simulink model "simulink_main"  (R2020b)
settings: Solver=FixedStepAuto  StartTime=0.0  StopTime=simTime  FixedStep=simulationStepTime  MaxStep=simulationStepTime  RelTol=1e-3
values from neighbouring files (symbols this model uses):
  link1MaxThreshold = 0    [main_CDTA.m]
  link1MinThreshold = 1    [main_CDTA.m]
undefined symbols (not defined in the file or in its folder): delayCPE1Controller1, delayCPE2Controller1, processingTimeCPEUpdate, processTimeController1, processTimeCPE1MonitoringInfo
settings Model: Creator=carmi  LastModifiedBy=carmi
settings DataIOCC: LimitDataPoints=on  SaveOutput=off  SaveTime=off  ReturnWorkspaceOutputs=off
settings OptimizationCC: BooleanDataType=off  DefaultParameterBehavior=Inlined  LocalBlockOutputs=off  LifeSpan=inf
settings DebuggingCC: AlgebraicLoopMsg=error  SingleTaskRateTransMsg=error  AllowSymbolicDim=off  SFUnexpectedBacktrackingDiag=warning  SFNoUnconditionalDefaultTransitionDiag=warning  SFExecutionAtInitializationDiag=none  ArithmeticOperatorsInVariantConditions=warning
settings SFSimCC: SimUseLocalCustomCode=off  CustomCodeUndefinedFunction=UseInterfaceOnly
settings RTWCC: RTWUseLocalCustomCode=off
settings CodeAppCC: StateflowObjectComments=on
settings GRTTargetCC: TargetLangStandard=C89/C90 (ANSI)
settings ConfigComp: CovMetricSettings=dw  CovSaveCumulativeToWorkspaceVar=on  CovSaveSingleToWorkspaceVar=on  CovExternalEMLEnable=off  CovSFcnEnable=off

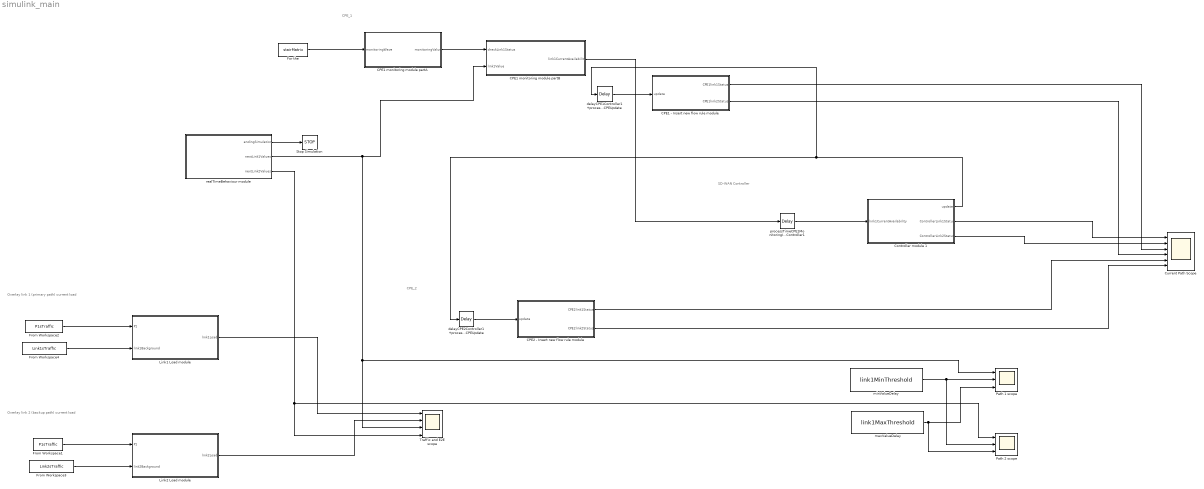
== system simulink_main ==
  note: SD-WAN Controller
  note: Overlay link 2 (backup path) current load
  note: CPE_1
  note: CPE_2
  note: Overlay link 1 (primary path) current load
  CPE1 - Insert new flow rule module : MATLAB Function  TreatAsAtomicUnit=on
  CPE1 monitoring module partA : MATLAB Function  TreatAsAtomicUnit=on
  CPE1 monitoring module partB : MATLAB Function  TreatAsAtomicUnit=on
  CPE2 - Insert new flow rule module : MATLAB Function  TreatAsAtomicUnit=on
  "Controller module 1 " : MATLAB Function  TreatAsAtomicUnit=on
  Current Path Scope : Scope  NumInputPorts=6
  For the : FromWorkspace  VariableName=stairMatrix  OutputAfterFinalValue=Setting to zero
  From Workspace1 : FromWorkspace  VariableName=P1sTraffic  OutputAfterFinalValue=Setting to zero
  From Workspace2 : FromWorkspace  VariableName=P1sTraffic  OutputAfterFinalValue=Setting to zero
  From Workspace3 : FromWorkspace  VariableName=Link2sTraffic  OutputAfterFinalValue=Setting to zero
  From Workspace4 : FromWorkspace  VariableName=Link1sTraffic  OutputAfterFinalValue=Setting to zero
  Link1 Load module : MATLAB Function  TreatAsAtomicUnit=on
  Link2 Load module : MATLAB Function  TreatAsAtomicUnit=on
  Path 1 scope : Scope  NumInputPorts=3
  Path 2 scope : Scope  NumInputPorts=3
  Stop Simulation : Stop
  Traffic and E2E scope : Scope  NumInputPorts=4
  delayCPE1Controller1+processingTimeCPEUpdate : TransportDelay  DelayTime=delayCPE1Controller1+processingTimeCPEUpdate
  delayCPE2Controller1+processingTimeCPEUpdate : TransportDelay  DelayTime=delayCPE2Controller1+processingTimeCPEUpdate
  maxValueDelay : Constant  Value=link1MaxThreshold
  minValueDelay : Constant  Value=link1MinThreshold
  processTimeCPE1MonitoringInfo+delayCPE1Controller1+processTimeController1 : TransportDelay  DelayTime=processTimeCPE1MonitoringInfo+delayCPE1Controller1+processTimeController1  InitialOutput=-1
  realTimeBehaviour module : MATLAB Function  TreatAsAtomicUnit=on
  wires:
  CPE1 monitoring module partB/1(link1CurrentAvailability) -> processTimeCPE1MonitoringInfo+delayCPE1Controller1+processTimeController1/1
  processTimeCPE1MonitoringInfo+delayCPE1Controller1+processTimeController1/1 -> "Controller module 1 "/1(link1CurrentAvailability)
  delayCPE2Controller1+processingTimeCPEUpdate/1 -> CPE2 - Insert new flow rule module/1(update)
  delayCPE1Controller1+processingTimeCPEUpdate/1 -> CPE1 - Insert new flow rule module/1(update)
  From Workspace3/1 -> Link2 Load module/2(link2Background)
  From Workspace1/1 -> Link2 Load module/1(P1)
  CPE1 monitoring module partA/1(monitoringValue) -> CPE1 monitoring module partB/1(checkLink1Status)
  "Controller module 1 "/1(update) -> delayCPE1Controller1+processingTimeCPEUpdate/1, delayCPE2Controller1+processingTimeCPEUpdate/1
  For the/1 -> CPE1 monitoring module partA/1(monitoringWave)
  realTimeBehaviour module/1(endingSimulation) -> Stop Simulation/1
  realTimeBehaviour module/2(nextLink1Values) -> Traffic and E2E scope/3, Path 1 scope/1, CPE1 monitoring module partB/2(link1Value)
  CPE2 - Insert new flow rule module/1(CPE2link1Status) -> Current Path Scope/5
  CPE2 - Insert new flow rule module/2(CPE2link2Status) -> Current Path Scope/6
  "Controller module 1 "/2(ControllerLink1Status) -> Current Path Scope/1
  "Controller module 1 "/3(ControllerLink2Status) -> Current Path Scope/2
  CPE1 - Insert new flow rule module/1(CPE1link1Status) -> Current Path Scope/3
  CPE1 - Insert new flow rule module/2(CPE1link2Status) -> Current Path Scope/4
  Link2 Load module/1(link2Load) -> Traffic and E2E scope/2
  realTimeBehaviour module/3(nextLink2Values) -> Path 2 scope/1, Traffic and E2E scope/4
  From Workspace4/1 -> Link1 Load module/2(link1Background)
  Link1 Load module/1(link1Load) -> Traffic and E2E scope/1
  From Workspace2/1 -> Link1 Load module/1(P1)
  minValueDelay/1 -> Path 2 scope/2, Path 1 scope/2
  maxValueDelay/1 -> Path 2 scope/3, Path 1 scope/3

== matlab function simulink_main/Controller module 1  ==
  data: link1CurrentAvailability input; update output; ControllerLink1Status output; ControllerLink2Status output
function [update,ControllerLink1Status, ControllerLink2Status] = pathComputation(link1CurrentAvailability)
    coder.extrinsic('evalin', 'assignin');  
    ControllerLink1Status=0; 
    ControllerLink1Status= evalin('base','ControllerLink1Status'); 
    ControllerLink2Status=0; 
    ControllerLink2Status= evalin('base','ControllerLink2Status'); 
    link1Behaviour=0;
    link1Behaviour=evalin('base','link1Behaviour');    
    link1Behaviour = 0;
    link1Behaviour = evalin('base','link1Behaviour');
    minValueDelay=0;
    minValueDelay=evalin('base','link1MinThreshold');
    maxValueDelay=0; 
    maxValueDelay=evalin('base','link1MaxThreshold');
    thresholdType=0; 
    thresholdType = evalin('base','thresholdType');

    if link1Behaviour==1 
        link1CurrentAvailability=round(link1CurrentAvailability); 
    end
        link1ReRoutingProcedure=0;
        update=0;       
        link2ReRoutingProcedure=0;
           if(link1CurrentAvailability~=-1 )                
                link1ReRoutingProcedure=evalin('base','link1ReRoutingProcedure'); 
                link2ReRoutingProcedure=evalin('base','link2ReRoutingProcedure'); 
                if(~isnan(link1CurrentAvailability)) 
                    checkLink1=false; 
                    if (link1Behaviour==1)
                        if(link1CurrentAvailability==maxValueDelay) 
                           checkLink1=true;
                        end
                    else
                        if(link1CurrentAvailability>=maxValueDelay)
                            checkLink1=true;
                        end
                    end
                    
                    if(checkLink1==true) 
                        if(ControllerLink2Status==0)              
                            if(link2ReRoutingProcedure==0)
                                assignin('base','ControllerLink1Status',0); 
                                assignin('base','ControllerLink2Status',1);  
                                assignin('base','link1ReRoutingProcedure',2);  
                                ControllerLink1Status= evalin('base','ControllerLink1Status'); 
                                ControllerLink2Status= evalin('base','ControllerLink2Status');
                                link1ReRoutingProcedure= evalin('base','link1ReRoutingProcedure');
                                update=1;
                            else
                                fprintf("");  
                            end
                        else
                            fprintf("");
                        end
                    else  
                        if (ControllerLink1Status==0)  
                            if(link1ReRoutingProcedure==0)
                               if(thresholdType==1 || (thresholdType==2 && link1CurrentAvailability<minValueDelay && link1CurrentAvailability>0) ) 
                                    assignin('base','ControllerLink2Status',0);
                                    assignin('base','ControllerLink1Status',1);  
                                    assignin('base','link2ReRoutingProcedure',2);
                                    update=1;
                                    ControllerLink1Status= evalin('base','ControllerLink1Status');
                                    ControllerLink2Status= evalin('base','ControllerLink2Status');
                                    link2ReRoutingProcedure= evalin('base','link2ReRoutingProcedure');
                                else
                                    fprintf("");    
                                end
                            else
                                fprintf(""); 
                            end
                        else
                            fprintf("");
                        end
                    end
                else
                    fprintf("Measurement is NaN \n");          
                end   
           end       
end

== matlab function simulink_main/CPE1 monitoring module partB ==
  data: checkLink1Status input; link1Value input; link1CurrentAvailability output
function link1CurrentAvailability = sendMonitoringInfoToController1(checkLink1Status,link1Value)
    link1CurrentAvailability=-1;    
    checkLink1Status=floor(checkLink1Status); 
    if(checkLink1Status==1) 
        link1CurrentAvailability=link1Value;
    end   
end

== matlab function simulink_main/CPE2 - Insert new flow rule module ==
  data: update input; CPE2link1Status output; CPE2link2Status output
function [CPE2link1Status, CPE2link2Status] = updatePath(update)
    coder.extrinsic('evalin', 'assignin'); 
    CPE2link1Status=0; 
    CPE2link1Status= evalin('base','CPE2link1Status'); 
    CPE2link2Status=0; 
    CPE2link2Status= evalin('base','CPE2link2Status');     
    link1ReRoutingProcedure=0; 
    link1ReRoutingProcedure= evalin('base','link1ReRoutingProcedure'); 
    link2ReRoutingProcedure=0; 
    link2ReRoutingProcedure= evalin('base','link2ReRoutingProcedure');    
    update=round(update);
    if(update<=0.5)     
        fprintf("");
    else
        if(link1ReRoutingProcedure>0) 
           if(CPE2link2Status==0)
                assignin('base','CPE2link1Status',0);
                assignin('base','CPE2link2Status',1);         
                assignin('base','link1ReRoutingProcedure',link1ReRoutingProcedure-1); 
                CPE2link2Status= evalin('base','CPE2link2Status');
                CPE2link1Status= evalin('base','CPE2link1Status');
            else
                fprintf("");
            end
        else
            if(link2ReRoutingProcedure>0)
                if(CPE2link1Status==0)
                    assignin('base','CPE2link2Status',0);
                    assignin('base','CPE2link1Status',1);
                    assignin('base','link2ReRoutingProcedure',link2ReRoutingProcedure-1);
                    CPE2link2Status= evalin('base','CPE2link2Status');
                    CPE2link1Status= evalin('base','CPE2link1Status');
                else
                    fprintf("");
                end
            end
        end
    end   
end

== matlab function simulink_main/CPE1 - Insert new flow rule module ==
  data: update input; CPE1link1Status output; CPE1link2Status output
function [CPE1link1Status,CPE1link2Status] = updatePath(update)
    coder.extrinsic('evalin', 'assignin'); 
    CPE1link1Status=0; 
    CPE1link1Status= evalin('base','CPE1link1Status'); 
    CPE1link2Status=0; 
    CPE1link2Status= evalin('base','CPE1link2Status'); 
    numberOfReroutings=0;
    numberOfReroutings=evalin('base','numberOfReroutings');
    link1ReRoutingProcedure=0; 
    link1ReRoutingProcedure= evalin('base','link1ReRoutingProcedure'); 
    link2ReRoutingProcedure=0; 
    link2ReRoutingProcedure= evalin('base','link2ReRoutingProcedure');     
    update=round(update); 
    if(update<=0.5 )  
        fprintf("  "); 
    else
        
        if(link1ReRoutingProcedure>0) 
            if(CPE1link2Status==0)
                assignin('base','CPE1link1Status',0);
                assignin('base','CPE1link2Status',1);          
                assignin('base','link1ReRoutingProcedure',link1ReRoutingProcedure-1);
                CPE1link2Status= evalin('base','CPE1link2Status');
                CPE1link1Status= evalin('base','CPE1link1Status');
                numberOfReroutings=numberOfReroutings+1;
            else
                fprintf("");
            end
        else
            if(link2ReRoutingProcedure>0)
                if(CPE1link1Status==0)
                    assignin('base','CPE1link2Status',0);
                    assignin('base','CPE1link1Status',1);
                    assignin('base','link2ReRoutingProcedure',link2ReRoutingProcedure-1);
                    CPE1link2Status= evalin('base','CPE1link2Status');
                    CPE1link1Status= evalin('base','CPE1link1Status');
                    numberOfReroutings=numberOfReroutings+1;
                else
                     fprintf("");
                end
            end
        end
    end
    assignin('base','numberOfReroutings',numberOfReroutings);   
end

== matlab function simulink_main/Link1 Load module ==
  data: P1 input; link1Load output; link1Background input
function link1Load = evaluateLink1CurrentLoad(P1,link1Background)
    coder.extrinsic('evalin', 'assignin');  
    ControllerLink1Status=0;
    ControllerLink1Status= evalin('base','ControllerLink1Status'); 
    CPE1link1Status=0;
    CPE1link1Status=evalin('base','CPE1link1Status'); 
    CPE2link1Status=0;
    CPE2link1Status = evalin('base','CPE2link1Status'); 
    link1Load=link1Background;
    if(ControllerLink1Status==1) 
        if(CPE1link1Status==1 && CPE2link1Status==1)
            link1Load=P1+link1Load;
        end
    end
end

== matlab function simulink_main/CPE1 monitoring module partA ==
  data: monitoringWave input; monitoringValue output
function monitoringValue = defineMonitoringFunction(monitoringWave)  
    monitoringValue=floor(monitoringWave); 
    if(monitoringWave>0.999)
         monitoringValue=1;
    end     
end

== matlab function simulink_main/Link2 Load module ==
  data: P1 input; link2Load output; link2Background input
function link2Load = evaluateLink2CurrentLoad(P1,link2Background)
    coder.extrinsic('evalin', 'assignin');  
    ControllerLink2Status=0;
    ControllerLink2Status= evalin('base','ControllerLink2Status'); 
    CPE1link2Status=0;
    CPE1link2Status=evalin('base','CPE1link2Status'); 
    CPE2link2Status=0;
    CPE2link2Status = evalin('base','CPE2link2Status'); 
    link2Load=link2Background;
    if(ControllerLink2Status==1)
        if(CPE1link2Status==1 && CPE2link2Status==1)
            link2Load=P1+link2Load;
        end
    end
end

== matlab function simulink_main/realTimeBehaviour module ==
  data: endingSimulation output; nextLink1Values output; nextLink2Values output
function [endingSimulation,nextLink1Values,nextLink2Values]=realTimeBehaviour()%[link1Delay,link2Delay] = computeLinksDelay()
    endingSimulation=0;
    nextLink1Values=0;
    nextLink2Values=0;
    coder.extrinsic('evalin', 'assignin');
    eml.extrinsic('checkCurrentLink');
    feval('checkCurrentLink');   
    index=0;
    index=evalin('base','index');
    timeInstants=0;
    timeInstants=evalin('base','timeInstants');
    typeOfAnalysis=0;
    typeOfAnalysis=evalin('base','typeOfAnalysis');
    eml.extrinsic('sensitivityRepetition');
    switch typeOfAnalysis
        case 1 %sensitivity            
            if(index~=timeInstants+1)
                feval('sensitivityRepetition');
            end 
    end    
    eml.extrinsic('convergenceRepetition');
    switch typeOfAnalysis
        case 2 %convergence
            if(index~=timeInstants+1)
                feval('convergenceRepetition');
            end       
    end    
    eml.extrinsic('dataPlane');
    feval('dataPlane');  
    eml.extrinsic('sensitivityRepetition');
    switch typeOfAnalysis
        case 1  %sensitivity 
            if(index==timeInstants+1)
                feval('sensitivityRepetition');
            end 
    end    
    eml.extrinsic('convergenceRepetition');
    switch typeOfAnalysis
        case 2 %convergence
            if(index==timeInstants+1)
                feval('convergenceRepetition');
            end       
    end        
    anticipateEnding=false;
    anticipateEnding=evalin('base','anticipateEndingSimulation');
    if anticipateEnding==true
        endingSimulation=1;
    end    
    valuesLink1Matrix=zeros(timeInstants+1,2);
    valuesLink1Matrix=evalin('base','valuesLink1Matrix');
    valuesLink2Matrix=zeros(timeInstants+1,2);
    valuesLink2Matrix=evalin('base','valuesLink2Matrix');    
    nextLink1Values=valuesLink1Matrix(index,2);
    nextLink2Values=valuesLink2Matrix(index,2);          
end
